simulink model "PWM"  (R2020b)
settings: Solver=VariableStepAuto  StartTime=0.0  StopTime=50  RelTol=1e-3
libraries: simulink x1
settings Model: Creator=99003727  LastModifiedBy=99003727

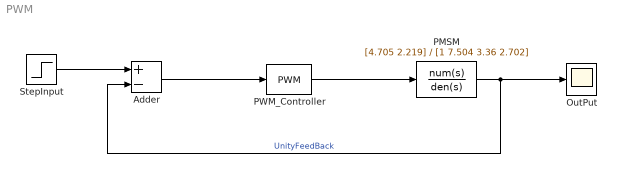
== system PWM ==
  Adder : Sum  Inputs=+-
  OutPut : Scope
  PMSM : TransferFcn  Numerator=[4.705 2.219]  Denominator=[1 7.504 3.36 2.702]
  PWM_Controller : simulink/Discontinuities/PWM  DisableCoverage=on  Period=0.1  DisallowZeroDutyCycle=off  RunAtFixedTimeIntervals=off  SampleTime=0.1
  StepInput : Step  Time=0  Before=1  SampleTime=0
  wires:
  StepInput/1 -> Adder/1
  Adder/1 -> PWM_Controller/1
  PWM_Controller/1 -> PMSM/1
  PMSM/1 -> OutPut/1, Adder/2  "UnityFeedBack"
